simulink model "Fuzzy_Control_Pendulum_Cau_1"  (Simulink 9.3)
settings: Solver=ode5  StartTime=0.0  StopTime=20  FixedStep=0.01  RelTol=1e-3  EnableMultiTasking=on
libraries: fuzblock x1
settings Model: Creator=lemin  LastModifiedBy=forev
settings DataIOCC: LimitDataPoints=on
settings OptimizationCC: ExpressionDepthLimit=2147483647
settings DebuggingCC: SolverPrmCheckMsg=warning  StateNameClashWarn=warning  SFExecutionAtInitializationDiag=warning
settings GRTTargetCC: GeneratePreprocessorConditionals=Disable all

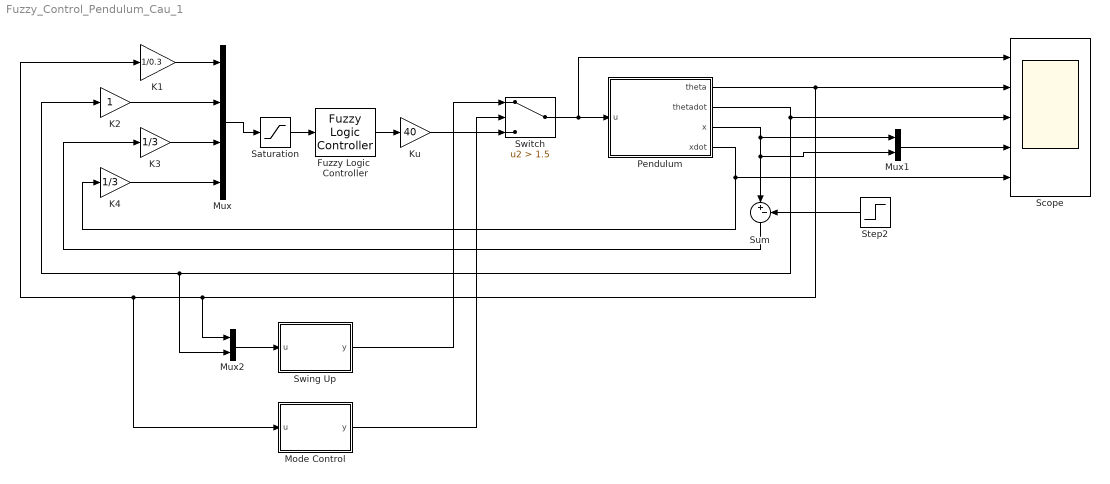
== system Fuzzy_Control_Pendulum_Cau_1 ==
  Fuzzy Logic  Controller : fuzblock/Fuzzy Logic  Controller  FIS='Pendulum.fis'  OutputSampleNumber=101  DataType=double  FuzzifiedInputs=off  RuleFiringStrengths=off  RuleOutputs=off  AggregatedOutputs=off  SimulateUsing=Interpreted execution  OutOfRangeInputValueMessage=warning  NoRuleFiredMessage=warning  EmptyOutputFuzzySetMessage=warning
  K1 : Gain  Gain=1/0.3
  K2 : Gain
  K3 : Gain  Gain=1/3
  K4 : Gain  Gain=1/3
  Ku : Gain  Gain=40
  Mode Control : MATLAB Function  TreatAsAtomicUnit=on
  Mux : Mux
  Mux1 : Mux  Inputs=2
  Mux2 : Mux  Inputs=2
  Pendulum : Subsystem  mask{p=1, m=0.1, l=0.5, g=9.81, thetadot0=pi, thetadot1=0, xdot0=0, xdot1=0}
      mask prompts: p "Khoi luong xe"; m "Khoi luong con lac"; l "Chieu dai day"; g "Gia toc trong truong"; thetadot0 "Initial theta"; thetadot1 "Initial thetadot"; xdot0 "Initial x"; xdot1 "Initial xdot"
  Saturation : Saturate  UpperLimit=1  LowerLimit=-1
  Scope : Scope  NumInputPorts=5
  Step2 : Step  Time=0  After=0  SampleTime=0.01
  Sum : Sum  Inputs=|+-
  Swing Up : MATLAB Function  TreatAsAtomicUnit=on
  Switch : Switch  Criteria=u2 > Threshold  Threshold=1.5
  wires:
  Fuzzy Logic  Controller/1 -> Ku/1
  Saturation/1 -> Fuzzy Logic  Controller/1
  Mux/1 -> Saturation/1
  Pendulum/2(thetadot) -> Mux2/2, K2/1, Scope/3
  K1/1 -> Mux/1
  K2/1 -> Mux/2
  K3/1 -> Mux/3
  K4/1 -> Mux/4
  Pendulum/3(x) -> Mux1/2, Sum/1, Mux1/1
  Sum/1 -> K3/1
  Pendulum/1(theta) -> Scope/2, Mode Control/1(u), K1/1, Mux2/1
  Mux1/1 -> Scope/4
  Mux2/1 -> Swing Up/1(u)
  Mode Control/1(y) -> Switch/2
  Switch/1 -> Scope/1, Pendulum/1(u)
  Ku/1 -> Switch/3
  Swing Up/1(y) -> Switch/1
  Pendulum/4(xdot) -> K4/1, Scope/5
  Step2/1 -> Sum/2

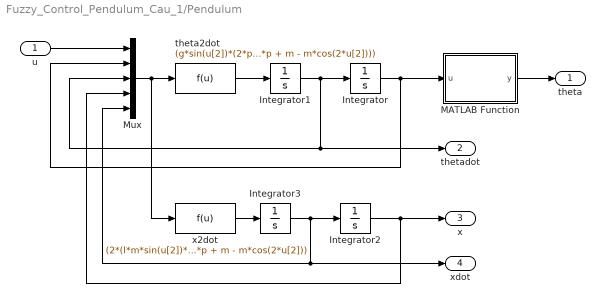
== system Fuzzy_Control_Pendulum_Cau_1/Pendulum ==
  u : Inport
  Integrator : Integrator  InitialCondition=thetadot0
  Integrator1 : Integrator  InitialCondition=thetadot1
  Integrator2 : Integrator  InitialCondition=xdot0
  Integrator3 : Integrator  InitialCondition=xdot1
  MATLAB Function : MATLAB Function  TreatAsAtomicUnit=on
  Mux : Mux  Inputs=5
  theta2dot : Fcn  Expr=(g*sin(u[2])*(2*p + 2*m))/(l*(2*p + m - m*cos(2*u[2]))) - (2*cos(u[2])*(l*m*sin(u[2])*u[3]^2 + u[1]))/(l*(2*p + m - m*cos(2*u[2])))
  x2dot : Fcn  Expr=(2*(l*m*sin(u[2])*u[3]^2 + u[1]))/(2*p + m - m*cos(2*u[2])) - (2*g*m*cos(u[2])*sin(u[2]))/(2*p + m - m*cos(2*u[2]))
  theta : Outport
  thetadot : Outport  Port=2
  x : Outport  Port=3
  xdot : Outport  Port=4
  wires:
  u/1 -> Mux/1
  Mux/1 -> theta2dot/1, x2dot/1
  theta2dot/1 -> Integrator1/1
  Integrator1/1 -> Integrator/1, Mux/3, thetadot/1
  Integrator/1 -> MATLAB Function/1(u), Mux/2
  x2dot/1 -> Integrator3/1
  Integrator3/1 -> Integrator2/1, Mux/5, xdot/1
  Integrator2/1 -> x/1, Mux/4
  MATLAB Function/1(y) -> theta/1

== matlab function Mode Control ==
  data: u input double; y output double
function y = fcn(u)
if (u>=-pi/6) && (u<=pi/6)
    y=1;
else
    y=2;
end
end

== matlab function Pendulum/MATLAB Function ==
  data: u input double; y output double
function y = fcn(u)
t = mod(u,2*pi);
if (t>pi)
    y=t-2*pi;
else
    y=t;
end
end

== matlab function Swing Up ==
  data: u input double; y output double
function y = fcn(u)
Usw =  4;
y = 0;
if (u(1) > 2*pi/3) && (u(1) <= pi) && (u(2) >= 0)
    y = Usw;
elseif (u(1) < -2*pi/3) && (u(1) >= -pi) && (u(2) <= 0)
    y = -Usw;
else
    y = 0;
end
end
